simulink model "MotorServo"  (R2021b)
settings: Solver=VariableStepAuto  StartTime=0.0  StopTime=10  RelTol=1e-3
settings Model: Creator=Attafahqi  LastModifiedBy=Attafahqi

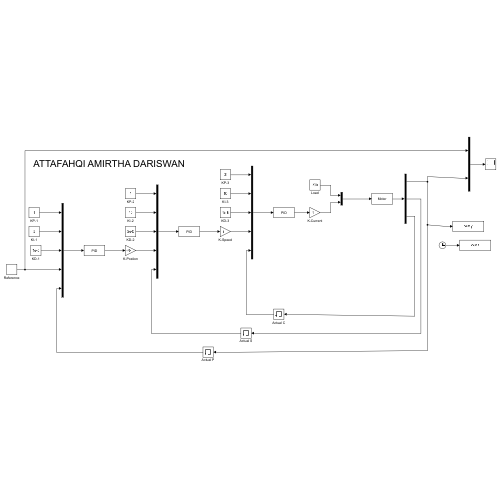
[thumbnail: Simulink's stored preview of the top-level diagram]
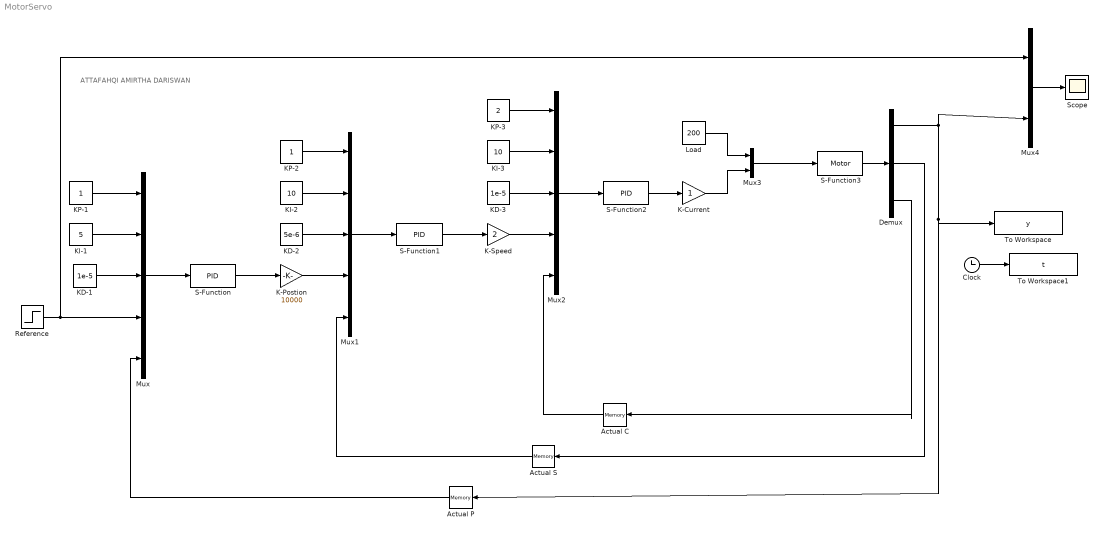
== system MotorServo ==
  note: ATTAFAHQI AMIRTHA DARISWAN
  Actual C : Memory
  Actual P : Memory
  Actual S : Memory
  Clock : Clock
  Demux : Demux  Outputs=3
  K-Current : Gain
  K-Postion : Gain  Gain=10000
  K-Speed : Gain  Gain=2
  KD-1 : Constant  Value=1e-5
  KD-2 : Constant  Value=5e-6
  KD-3 : Constant  Value=1e-5
  KI-1 : Constant  Value=5
  KI-2 : Constant  Value=10
  KI-3 : Constant  Value=10
  KP-1 : Constant
  KP-2 : Constant
  KP-3 : Constant  Value=2
  Load : Constant  Value=200
  Mux : Mux  Inputs=5
  Mux1 : Mux  Inputs=5
  Mux2 : Mux  Inputs=5
  Mux3 : Mux  Inputs=2
  Mux4 : Mux  Inputs=2
  Reference : Step  After=5  SampleTime=0
  S-Function : S-Function  FunctionName=PID  SFunctionDeploymentMode=off  EnableBusSupport=off
  S-Function1 : S-Function  FunctionName=PID  SFunctionDeploymentMode=off  EnableBusSupport=off
  S-Function2 : S-Function  FunctionName=PID  SFunctionDeploymentMode=off  EnableBusSupport=off
  S-Function3 : S-Function  FunctionName=Motor  SFunctionDeploymentMode=off  EnableBusSupport=off
  Scope : Scope
  To Workspace : ToWorkspace  VariableName=y  SampleTime=-1
  To Workspace1 : ToWorkspace  VariableName=t  SaveFormat=Timeseries  SampleTime=-1
  wires:
  Mux/1 -> S-Function/1
  S-Function/1 -> K-Postion/1
  Mux1/1 -> S-Function1/1
  S-Function1/1 -> K-Speed/1
  Mux2/1 -> S-Function2/1
  S-Function2/1 -> K-Current/1
  K-Speed/1 -> Mux2/4
  K-Postion/1 -> Mux1/4
  KP-1/1 -> Mux/1
  KD-1/1 -> Mux/3
  KI-1/1 -> Mux/2
  KP-2/1 -> Mux1/1
  KI-2/1 -> Mux1/2
  KD-2/1 -> Mux1/3
  KP-3/1 -> Mux2/1
  KI-3/1 -> Mux2/2
  KD-3/1 -> Mux2/3
  Actual C/1 -> Mux2/5
  Actual S/1 -> Mux1/5
  Actual P/1 -> Mux/5
  Mux4/1 -> Scope/1
  Mux3/1 -> S-Function3/1
  K-Current/1 -> Mux3/2
  Load/1 -> Mux3/1
  Clock/1 -> To Workspace1/1
  S-Function3/1 -> Demux/1
  Demux/3 -> Actual C/1
  Demux/2 -> Actual S/1
  Demux/1 -> To Workspace/1, Actual P/1, Mux4/2
  Reference/1 -> Mux4/1, Mux/4
